simulink model "QuadArchitecture"  (R2026a)
settings: configuration reference "quad_config" (kept outside this file)
settings Model: DataDictionary=QuadData.sldd  PacingRate=4  Creator=The MathWorks, Inc.  LastModifiedBy=The MathWorks, Inc.
settings ConfigSetRef: SourceName=quad_config

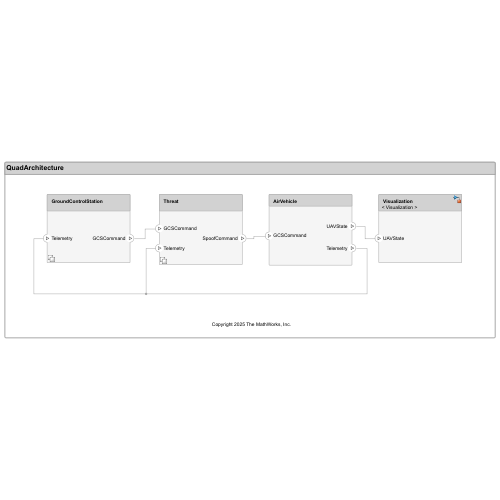
[thumbnail: Simulink's stored preview of the top-level diagram]
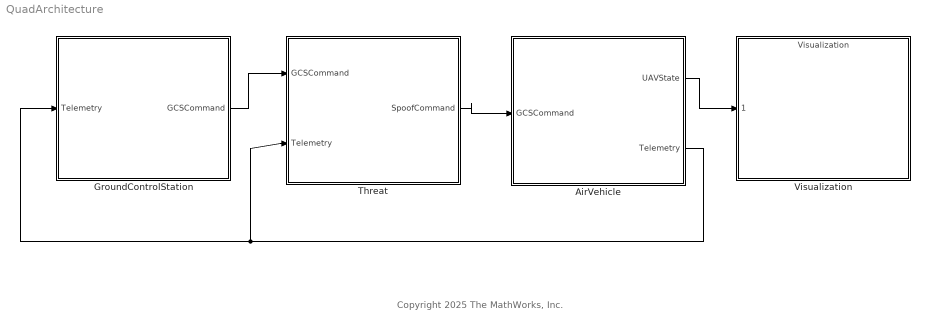
== system QuadArchitecture ==
  note: Copyright 2025 The MathWorks, Inc.
  AirVehicle : Subsystem
      settings: PortSchema="{\"entries\":[{\"content\":{\"headerSize\":26,\"margin\":15,\"minimumSpacing\":25,\"sides\":[{\"content\":{\"connectorIds\":[\"In1\"]},\"type\":\"ConnectorPlacement.EquallySpacedRectSide\",\"uuid\":\"972de20d-f328-4fd0-89f5-295843657512\"},{\"content\":{\"connectorIds\":[\"Out2\",\"Out1\"],\"side\":\"RIGHT\"},\"type\":\"ConnectorPlacement.EquallySpacedRectSide\",\"uuid\":\"134439da-fb85-42f0-a6e3-e26c335dbcbe\"},{\"content\":{\"side\":\"TOP\"},\"type\":\"ConnectorPlacement.EquallySpacedRectSide\",\"uuid\":\"868b2dd7-5d80-431a-bb16-a2f793ede056\"}]},\"type\":\"ConnectorPlacement.EquallySpacedConnector\",\"uuid\":\"adddc505-6cbf-480f-b95d-01cd6e84ae8d\"}],\"packageUris\":[\"http://schema.mathworks.com/mf0/Connector/R2020b\"],\"version\":\"1.0\"}"
  GroundControlStation : Subsystem  Variant=on  VariantControl=Choice
      settings: PortSchema="{\"entries\":[{\"content\":{\"headerSize\":38,\"margin\":15,\"minimumSpacing\":25,\"sides\":[{\"content\":{\"connectorIds\":[\"In1\"]},\"type\":\"ConnectorPlacement.EquallySpacedRectSide\",\"uuid\":\"7662a576-a240-432d-97be-55e19f57859a\"},{\"content\":{\"connectorIds\":[\"Out1\"],\"side\":\"RIGHT\"},\"type\":\"ConnectorPlacement.EquallySpacedRectSide\",\"uuid\":\"93b9fbbc-f8c4-4932-b9bb-3841cff066c6\"},{\"content\":{\"connectorIds\":[],\"side\":\"TOP\"},\"type\":\"ConnectorPlacement.EquallySpacedRectSide\",\"uuid\":\"5bdbe3e7-55b6-4275-a555-da2f215fbbe6\"}]},\"type\":\"ConnectorPlacement.EquallySpacedConnector\",\"uuid\":\"7fdcb0bb-8d60-4179-a2fb-32da7250d2ba\"}],\"packageUris\":[\"http://schema.mathworks.com/mf0/Connector/R2020b\"],\"version\":\"1.0\"}"
  Threat : Subsystem  Variant=on  VariantControl=Choice
      settings: PortSchema="{\"entries\":[{\"content\":{\"headerSize\":38,\"margin\":15,\"minimumSpacing\":25,\"sides\":[{\"content\":{\"connectorIds\":[\"In1\",\"In2\"]},\"type\":\"ConnectorPlacement.EquallySpacedRectSide\",\"uuid\":\"972de20d-f328-4fd0-89f5-295843657512\"},{\"content\":{\"connectorIds\":[\"Out1\"],\"side\":\"RIGHT\"},\"type\":\"ConnectorPlacement.EquallySpacedRectSide\",\"uuid\":\"134439da-fb85-42f0-a6e3-e26c335dbcbe\"},{\"content\":{\"side\":\"TOP\"},\"type\":\"ConnectorPlacement.EquallySpacedRectSide\",\"uuid\":\"868b2dd7-5d80-431a-bb16-a2f793ede056\"}]},\"type\":\"ConnectorPlacement.EquallySpacedConnector\",\"uuid\":\"adddc505-6cbf-480f-b95d-01cd6e84ae8d\"}],\"packageUris\":[\"http://schema.mathworks.com/mf0/Connector/R2020b\"],\"version\":\"1.0\"}"
  Visualization : ModelReference  ModelNameDialog=Visualization  SimulationMode=Normal  ModelReferenceVersion=11.4
      settings: PortSchema="{\"entries\":[{\"content\":{\"headerSize\":38,\"margin\":15,\"minimumSpacing\":25,\"sides\":[{\"content\":{\"connectorIds\":[\"In1\"]},\"type\":\"ConnectorPlacement.EquallySpacedRectSide\",\"uuid\":\"6721b7c2-8ab9-44e5-9ceb-8e1a3ee04589\"},{\"content\":{\"connectorIds\":[],\"side\":\"RIGHT\"},\"type\":\"ConnectorPlacement.EquallySpacedRectSide\",\"uuid\":\"3cd6ecf7-e51b-4f75-96cf-07e3d6ff229c\"},{\"content\":{\"connectorIds\":[],\"side\":\"TOP\"},\"type\":\"ConnectorPlacement.EquallySpacedRectSide\",\"uuid\":\"f91676ab-b0f6-405b-b8b9-c3171517e379\"}]},\"type\":\"ConnectorPlacement.EquallySpacedConnector\",\"uuid\":\"6f23ebeb-60da-469e-8f3b-5adae7c8af4f\"}],\"packageUris\":[\"http://schema.mathworks.com/mf0/Connector/R2020b\"],\"version\":\"1.0\"}"
  wires:
  AirVehicle/1(Telemetry) -> Threat/2(Telemetry), GroundControlStation/1(Telemetry)
  AirVehicle/2(UAVState) -> Visualization/1
  Threat/1(SpoofCommand) -> AirVehicle/1(GCSCommand)
  GroundControlStation/1(GCSCommand) -> Threat/1(GCSCommand)

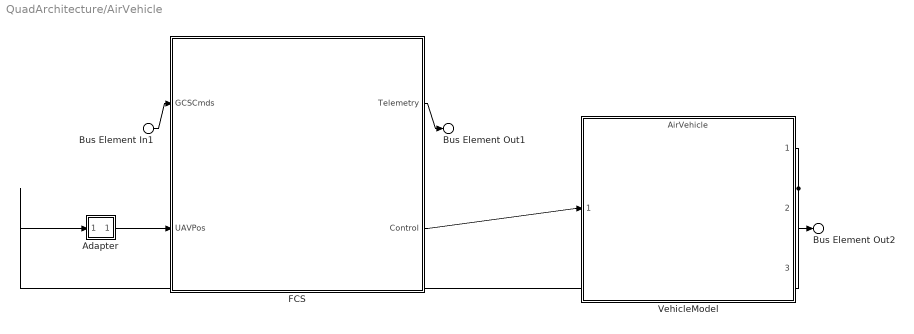
== system QuadArchitecture/AirVehicle ==
  Bus Element In1 : Inport  PortName=GCSCommand
  Adapter : Subsystem
      settings: PortSchema="{\"entries\":[{\"content\":{\"margin\":10,\"minimumSpacing\":15,\"sides\":[{\"content\":{\"connectorIds\":[\"In1\"]},\"type\":\"ConnectorPlacement.EquallySpacedRectSide\",\"uuid\":\"a2fff1cd-0e13-4741-b0cf-ef553acfd516\"},{\"content\":{\"connectorIds\":[\"Out1\"],\"side\":\"RIGHT\"},\"type\":\"ConnectorPlacement.EquallySpacedRectSide\",\"uuid\":\"37e44836-fd51-4d84-80b7-9025c833adfd\"},{\"content\":{\"connectorIds\":[],\"side\":\"TOP\"},\"type\":\"ConnectorPlacement.EquallySpacedRectSide\",\"uuid\":\"e6edc5e9-901f-4b36-8f7f-d0a35232da3b\"}]},\"type\":\"ConnectorPlacement.EquallySpacedConnector\",\"uuid\":\"83782042-2650-4988-9c4a-c1150f20d034\"}],\"packageUris\":[\"http://schema.mathworks.com/mf0/Connector/R2020b\"],\"version\":\"1.0\"}"
  FCS : Subsystem
      settings: PortSchema="{\"entries\":[{\"content\":{\"headerSize\":26,\"margin\":15,\"minimumSpacing\":25,\"sides\":[{\"content\":{\"connectorIds\":[\"In1\",\"In2\"]},\"type\":\"ConnectorPlacement.EquallySpacedRectSide\",\"uuid\":\"c19c5851-94a8-41ae-97b5-784b7360f27c\"},{\"content\":{\"connectorIds\":[\"Out1\",\"Out2\"],\"side\":\"RIGHT\"},\"type\":\"ConnectorPlacement.EquallySpacedRectSide\",\"uuid\":\"5a0e265f-6421-459c-9b38-1ace018e6962\"},{\"content\":{\"side\":\"TOP\"},\"type\":\"ConnectorPlacement.EquallySpacedRectSide\",\"uuid\":\"afc92b11-75c7-4a4a-94ab-c0816f6717ed\"}]},\"type\":\"ConnectorPlacement.EquallySpacedConnector\",\"uuid\":\"e74c21e7-420a-47a8-adb7-493ac11b1149\"}],\"packageUris\":[\"http://schema.mathworks.com/mf0/Connector/R2020b\"],\"version\":\"1.0\"}"
  VehicleModel : ModelReference  ModelNameDialog=AirVehicle  ModelReferenceVersion=12.4
      settings: PortSchema="{\"entries\":[{\"content\":{\"headerSize\":38,\"margin\":15,\"minimumSpacing\":25,\"sides\":[{\"content\":{\"connectorIds\":[\"In1\"]},\"type\":\"ConnectorPlacement.EquallySpacedRectSide\",\"uuid\":\"972de20d-f328-4fd0-89f5-295843657512\"},{\"content\":{\"connectorIds\":[\"Out1\",\"Out2\",\"Out3\"],\"side\":\"RIGHT\"},\"type\":\"ConnectorPlacement.EquallySpacedRectSide\",\"uuid\":\"134439da-fb85-42f0-a6e3-e26c335dbcbe\"},{\"content\":{\"side\":\"TOP\"},\"type\":\"ConnectorPlacement.EquallySpacedRectSide\",\"uuid\":\"868b2dd7-5d80-431a-bb16-a2f793ede056\"}]},\"type\":\"ConnectorPlacement.EquallySpacedConnector\",\"uuid\":\"adddc505-6cbf-480f-b95d-01cd6e84ae8d\"}],\"packageUris\":[\"http://schema.mathworks.com/mf0/Connector/R2020b\"],\"version\":\"1.0\"}"
  Bus Element Out1 : Outport  PortName=Telemetry
  Bus Element Out2 : Outport  Port=2  PortName=UAVState
  wires:
  FCS/1(Telemetry) -> Bus Element Out1/1
  VehicleModel/1 -> Bus Element Out2/1, Adapter/1(In)
  FCS/2(Control) -> VehicleModel/1
  Adapter/1(UAVPos) -> FCS/2(UAVPos)
  Bus Element In1/1 -> FCS/1(GCSCmds)

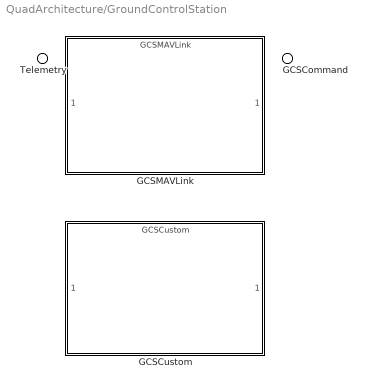
== system QuadArchitecture/GroundControlStation ==
  Telemetry : Inport
  GCSCustom : ModelReference  ModelNameDialog=GCSCustom  SimulationMode=Normal  VariantControl=varComms == 2  ModelReferenceVersion=12.2
      settings: PortSchema="{\"entries\":[{\"content\":{\"headerSize\":38,\"margin\":15,\"minimumSpacing\":25,\"sides\":[{\"content\":{\"connectorIds\":[\"In1\"]},\"type\":\"ConnectorPlacement.EquallySpacedRectSide\",\"uuid\":\"972de20d-f328-4fd0-89f5-295843657512\"},{\"content\":{\"connectorIds\":[\"Out1\"],\"side\":\"RIGHT\"},\"type\":\"ConnectorPlacement.EquallySpacedRectSide\",\"uuid\":\"134439da-fb85-42f0-a6e3-e26c335dbcbe\"},{\"content\":{\"connectorIds\":[],\"side\":\"TOP\"},\"type\":\"ConnectorPlacement.EquallySpacedRectSide\",\"uuid\":\"868b2dd7-5d80-431a-bb16-a2f793ede056\"}]},\"type\":\"ConnectorPlacement.EquallySpacedConnector\",\"uuid\":\"adddc505-6cbf-480f-b95d-01cd6e84ae8d\"}],\"packageUris\":[\"http://schema.mathworks.com/mf0/Connector/R2020b\"],\"version\":\"1.0\"}"
  GCSMAVLink : ModelReference  ModelNameDialog=GCSMAVLink  SimulationMode=Normal  VariantControl=varComms == 1  ModelReferenceVersion=12.4
      settings: PortSchema="{\"entries\":[{\"content\":{\"headerSize\":38,\"margin\":15,\"minimumSpacing\":25,\"sides\":[{\"content\":{\"connectorIds\":[\"In1\"]},\"type\":\"ConnectorPlacement.EquallySpacedRectSide\",\"uuid\":\"7662a576-a240-432d-97be-55e19f57859a\"},{\"content\":{\"connectorIds\":[\"Out1\"],\"side\":\"RIGHT\"},\"type\":\"ConnectorPlacement.EquallySpacedRectSide\",\"uuid\":\"93b9fbbc-f8c4-4932-b9bb-3841cff066c6\"},{\"content\":{\"connectorIds\":[],\"side\":\"TOP\"},\"type\":\"ConnectorPlacement.EquallySpacedRectSide\",\"uuid\":\"5bdbe3e7-55b6-4275-a555-da2f215fbbe6\"}]},\"type\":\"ConnectorPlacement.EquallySpacedConnector\",\"uuid\":\"7fdcb0bb-8d60-4179-a2fb-32da7250d2ba\"}],\"packageUris\":[\"http://schema.mathworks.com/mf0/Connector/R2020b\"],\"version\":\"1.0\"}"
  GCSCommand : Outport  OutDataTypeStr=Bus: GCSCmds

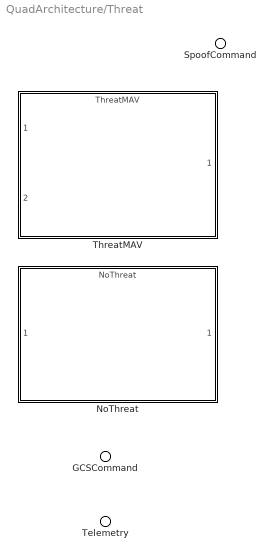
== system QuadArchitecture/Threat ==
  GCSCommand : Inport
  Telemetry : Inport  Port=2
  NoThreat : ModelReference  ModelNameDialog=NoThreat  SimulationMode=Normal  VariantControl=varThreat == 0  ModelReferenceVersion=2.0
      settings: PortSchema="{\"entries\":[{\"content\":{\"headerSize\":38,\"margin\":15,\"minimumSpacing\":25,\"sides\":[{\"content\":{\"connectorIds\":[\"In1\"]},\"type\":\"ConnectorPlacement.EquallySpacedRectSide\",\"uuid\":\"e9d8ad3e-caa9-432a-b411-be5fd036b273\"},{\"content\":{\"connectorIds\":[\"Out1\"],\"side\":\"RIGHT\"},\"type\":\"ConnectorPlacement.EquallySpacedRectSide\",\"uuid\":\"3984a8dd-9d03-4219-b4db-e54bb042947b\"},{\"content\":{\"side\":\"TOP\"},\"type\":\"ConnectorPlacement.EquallySpacedRectSide\",\"uuid\":\"6391b23f-1c48-490d-9fba-fd835ec6a9a7\"}]},\"type\":\"ConnectorPlacement.EquallySpacedConnector\",\"uuid\":\"c696faa4-67d5-4608-8425-39d05734b4d9\"}],\"packageUris\":[\"http://schema.mathworks.com/mf0/Connector/R2020b\"],\"version\":\"1.0\"}"
  ThreatMAV : ModelReference  ModelNameDialog=ThreatMAV  SimulationMode=Normal  VariantControl=varThreat == 1  ModelReferenceVersion=12.4
      settings: PortSchema="{\"entries\":[{\"content\":{\"headerSize\":38,\"margin\":15,\"minimumSpacing\":25,\"sides\":[{\"content\":{\"connectorIds\":[\"In1\",\"In2\"]},\"type\":\"ConnectorPlacement.EquallySpacedRectSide\",\"uuid\":\"972de20d-f328-4fd0-89f5-295843657512\"},{\"content\":{\"connectorIds\":[\"Out1\"],\"side\":\"RIGHT\"},\"type\":\"ConnectorPlacement.EquallySpacedRectSide\",\"uuid\":\"134439da-fb85-42f0-a6e3-e26c335dbcbe\"},{\"content\":{\"connectorIds\":[],\"side\":\"TOP\"},\"type\":\"ConnectorPlacement.EquallySpacedRectSide\",\"uuid\":\"868b2dd7-5d80-431a-bb16-a2f793ede056\"}]},\"type\":\"ConnectorPlacement.EquallySpacedConnector\",\"uuid\":\"adddc505-6cbf-480f-b95d-01cd6e84ae8d\"}],\"packageUris\":[\"http://schema.mathworks.com/mf0/Connector/R2020b\"],\"version\":\"1.0\"}"
  SpoofCommand : Outport  OutDataTypeStr=Bus: GCSCmds

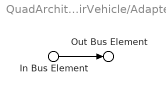
== system QuadArchitecture/AirVehicle/Adapter ==
  In Bus Element : Inport  PortName=In
  Out Bus Element : Outport  PortName=UAVPos
  wires:
  In Bus Element/1 -> Out Bus Element/1

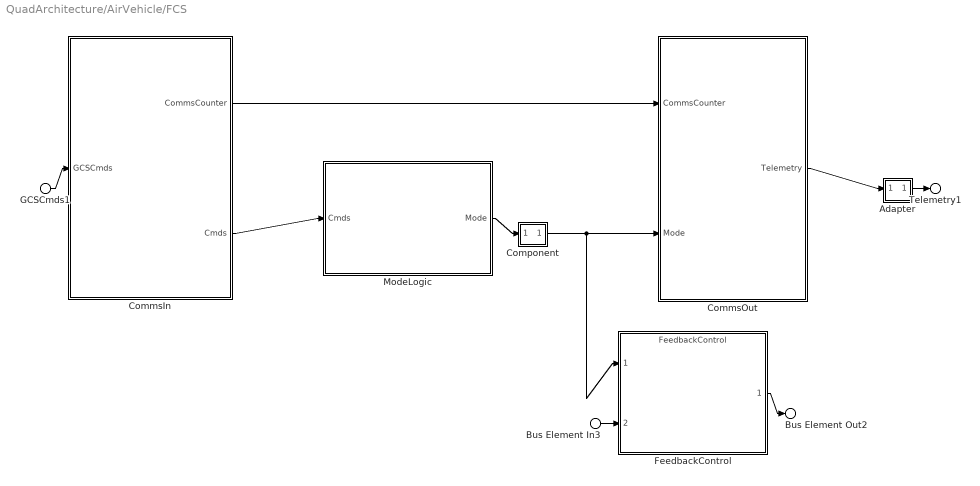
== system QuadArchitecture/AirVehicle/FCS ==
  GCSCmds1 : Inport  PortName=GCSCmds
  Bus Element In3 : Inport  Port=2  PortName=UAVPos
  Adapter : Subsystem
      settings: PortSchema="{\"entries\":[{\"content\":{\"margin\":10,\"minimumSpacing\":15,\"sides\":[{\"content\":{\"connectorIds\":[\"In1\"]},\"type\":\"ConnectorPlacement.EquallySpacedRectSide\",\"uuid\":\"54e91e87-63c7-4e3e-b7b9-664b6d97de79\"},{\"content\":{\"connectorIds\":[\"Out1\"],\"side\":\"RIGHT\"},\"type\":\"ConnectorPlacement.EquallySpacedRectSide\",\"uuid\":\"42371d78-e1ed-48f1-9b63-a93cba4f2c4a\"},{\"content\":{\"side\":\"TOP\"},\"type\":\"ConnectorPlacement.EquallySpacedRectSide\",\"uuid\":\"1916e499-1a19-4cfc-bc1b-e5fae3753eb5\"},{\"content\":{\"side\":\"BOTTOM\"},\"type\":\"ConnectorPlacement.EquallySpacedRectSide\",\"uuid\":\"be41fb80-b3af-48dd-88cd-2631e5331a74\"},{\"content\":{\"side\":\"HIDDEN\"},\"type\":\"ConnectorPlacement.EquallySpacedRectSide\",\"uuid\":\"3c256238-c293-40f1-b4b8-16721d7c0eb8\"}]},\"type\":\"ConnectorPlacement.EquallySpacedConnector\",\"uuid\":\"450fde28-8b10-4341-ad28-487e19ca1e28\"}],\"packageUris\":[\"http://schema.mathworks.com/mf0/Connector/R2020b\"],\"version\":\"1.0\"}"
  CommsIn : Subsystem  Variant=on  VariantControl=Choice
      settings: PortSchema="{\"entries\":[{\"content\":{\"headerSize\":38,\"margin\":15,\"minimumSpacing\":25,\"sides\":[{\"content\":{\"connectorIds\":[\"In1\"]},\"type\":\"ConnectorPlacement.EquallySpacedRectSide\",\"uuid\":\"972de20d-f328-4fd0-89f5-295843657512\"},{\"content\":{\"connectorIds\":[\"Out1\",\"Out2\"],\"side\":\"RIGHT\"},\"type\":\"ConnectorPlacement.EquallySpacedRectSide\",\"uuid\":\"134439da-fb85-42f0-a6e3-e26c335dbcbe\"},{\"content\":{\"connectorIds\":[],\"side\":\"TOP\"},\"type\":\"ConnectorPlacement.EquallySpacedRectSide\",\"uuid\":\"868b2dd7-5d80-431a-bb16-a2f793ede056\"}]},\"type\":\"ConnectorPlacement.EquallySpacedConnector\",\"uuid\":\"adddc505-6cbf-480f-b95d-01cd6e84ae8d\"}],\"packageUris\":[\"http://schema.mathworks.com/mf0/Connector/R2020b\"],\"version\":\"1.0\"}"
  CommsOut : Subsystem  Variant=on  VariantControl=Choice
      settings: PortSchema="{\"entries\":[{\"content\":{\"headerSize\":38,\"margin\":15,\"minimumSpacing\":25,\"sides\":[{\"content\":{\"connectorIds\":[\"In1\",\"In2\"]},\"type\":\"ConnectorPlacement.EquallySpacedRectSide\",\"uuid\":\"972de20d-f328-4fd0-89f5-295843657512\"},{\"content\":{\"connectorIds\":[\"Out1\"],\"side\":\"RIGHT\"},\"type\":\"ConnectorPlacement.EquallySpacedRectSide\",\"uuid\":\"134439da-fb85-42f0-a6e3-e26c335dbcbe\"},{\"content\":{\"connectorIds\":[],\"side\":\"TOP\"},\"type\":\"ConnectorPlacement.EquallySpacedRectSide\",\"uuid\":\"868b2dd7-5d80-431a-bb16-a2f793ede056\"}]},\"type\":\"ConnectorPlacement.EquallySpacedConnector\",\"uuid\":\"adddc505-6cbf-480f-b95d-01cd6e84ae8d\"}],\"packageUris\":[\"http://schema.mathworks.com/mf0/Connector/R2020b\"],\"version\":\"1.0\"}"
  Component : Subsystem
      settings: PortSchema="{\"entries\":[{\"content\":{\"margin\":10,\"minimumSpacing\":15,\"sides\":[{\"content\":{\"connectorIds\":[\"In1\"]},\"type\":\"ConnectorPlacement.EquallySpacedRectSide\",\"uuid\":\"17bee697-cd3a-4e06-942d-dac2ea0385a6\"},{\"content\":{\"connectorIds\":[\"Out1\"],\"side\":\"RIGHT\"},\"type\":\"ConnectorPlacement.EquallySpacedRectSide\",\"uuid\":\"6d1b1a8d-a046-48b6-94d3-1fa2831d6db3\"},{\"content\":{\"side\":\"TOP\"},\"type\":\"ConnectorPlacement.EquallySpacedRectSide\",\"uuid\":\"a053ff8f-e369-4dd3-abbb-f0419cd0218c\"}]},\"type\":\"ConnectorPlacement.EquallySpacedConnector\",\"uuid\":\"3ac54abc-4df1-48cf-8f38-e2b144d46944\"}],\"packageUris\":[\"http://schema.mathworks.com/mf0/Connector/R2020b\"],\"version\":\"1.0\"}"
  FeedbackControl : ModelReference  ModelNameDialog=FeedbackControl  SimulationMode=Normal  ModelReferenceVersion=8.3
      settings: PortSchema="{\"entries\":[{\"content\":{\"headerSize\":38,\"margin\":15,\"minimumSpacing\":25,\"sides\":[{\"content\":{\"connectorIds\":[\"In1\",\"In2\"]},\"type\":\"ConnectorPlacement.EquallySpacedRectSide\",\"uuid\":\"a2fff1cd-0e13-4741-b0cf-ef553acfd516\"},{\"content\":{\"connectorIds\":[\"Out1\"],\"side\":\"RIGHT\"},\"type\":\"ConnectorPlacement.EquallySpacedRectSide\",\"uuid\":\"37e44836-fd51-4d84-80b7-9025c833adfd\"},{\"content\":{\"side\":\"TOP\"},\"type\":\"ConnectorPlacement.EquallySpacedRectSide\",\"uuid\":\"e6edc5e9-901f-4b36-8f7f-d0a35232da3b\"}]},\"type\":\"ConnectorPlacement.EquallySpacedConnector\",\"uuid\":\"83782042-2650-4988-9c4a-c1150f20d034\"}],\"packageUris\":[\"http://schema.mathworks.com/mf0/Connector/R2020b\"],\"version\":\"1.0\"}"
  ModeLogic : Stateflow chart  TreatAsAtomicUnit=on
      settings: PortSchema="{\"entries\":[{\"content\":{\"headerSize\":26,\"margin\":15,\"minimumSpacing\":25,\"sides\":[{\"content\":{\"connectorIds\":[\"In1\"]},\"type\":\"ConnectorPlacement.EquallySpacedRectSide\",\"uuid\":\"a2fff1cd-0e13-4741-b0cf-ef553acfd516\"},{\"content\":{\"connectorIds\":[\"Out1\"],\"side\":\"RIGHT\"},\"type\":\"ConnectorPlacement.EquallySpacedRectSide\",\"uuid\":\"37e44836-fd51-4d84-80b7-9025c833adfd\"},{\"content\":{\"connectorIds\":[],\"side\":\"TOP\"},\"type\":\"ConnectorPlacement.EquallySpacedRectSide\",\"uuid\":\"e6edc5e9-901f-4b36-8f7f-d0a35232da3b\"}]},\"type\":\"ConnectorPlacement.EquallySpacedConnector\",\"uuid\":\"83782042-2650-4988-9c4a-c1150f20d034\"}],\"packageUris\":[\"http://schema.mathworks.com/mf0/Connector/R2020b\"],\"version\":\"1.0\"}"
  Telemetry1 : Outport  PortName=Telemetry
  Bus Element Out2 : Outport  Port=2  PortName=Control
  wires:
  CommsIn/1(CommsCounter) -> CommsOut/1(CommsCounter)
  CommsIn/2(Cmds) -> ModeLogic/1(Cmds)
  GCSCmds1/1 -> CommsIn/1(GCSCmds)
  FeedbackControl/1 -> Bus Element Out2/1
  Bus Element In3/1 -> FeedbackControl/2
  ModeLogic/1(Mode) -> Component/1(In)
  Component/1(Out) -> FeedbackControl/1, CommsOut/2(Mode)
  CommsOut/1(Telemetry) -> Adapter/1(TelemetryIn)
  Adapter/1(Telemetry) -> Telemetry1/1

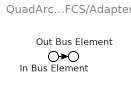
== system QuadArchitecture/AirVehicle/FCS/Adapter ==
  In Bus Element : Inport  PortName=TelemetryIn
  Out Bus Element : Outport  PortName=Telemetry
  wires:
  In Bus Element/1 -> Out Bus Element/1

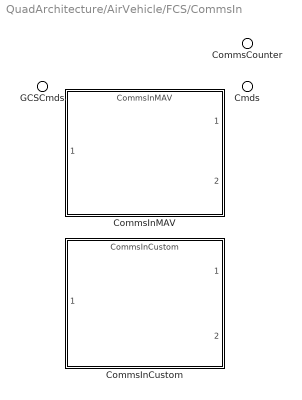
== system QuadArchitecture/AirVehicle/FCS/CommsIn ==
  GCSCmds : Inport  OutDataTypeStr=Bus: GCSCmds
  CommsInCustom : ModelReference  ModelNameDialog=CommsInCustom  SimulationMode=Normal  VariantControl=varComms == 2  ModelReferenceVersion=8.0
      settings: PortSchema="{\"entries\":[{\"content\":{\"headerSize\":38,\"margin\":15,\"minimumSpacing\":25,\"sides\":[{\"content\":{\"connectorIds\":[\"In1\"]},\"type\":\"ConnectorPlacement.EquallySpacedRectSide\",\"uuid\":\"972de20d-f328-4fd0-89f5-295843657512\"},{\"content\":{\"connectorIds\":[\"Out1\",\"Out2\"],\"side\":\"RIGHT\"},\"type\":\"ConnectorPlacement.EquallySpacedRectSide\",\"uuid\":\"134439da-fb85-42f0-a6e3-e26c335dbcbe\"},{\"content\":{\"connectorIds\":[],\"side\":\"TOP\"},\"type\":\"ConnectorPlacement.EquallySpacedRectSide\",\"uuid\":\"868b2dd7-5d80-431a-bb16-a2f793ede056\"}]},\"type\":\"ConnectorPlacement.EquallySpacedConnector\",\"uuid\":\"adddc505-6cbf-480f-b95d-01cd6e84ae8d\"}],\"packageUris\":[\"http://schema.mathworks.com/mf0/Connector/R2020b\"],\"version\":\"1.0\"}"
  CommsInMAV : ModelReference  ModelNameDialog=CommsInMAV  SimulationMode=Normal  VariantControl=varComms == 1  ModelReferenceVersion=8.1
      settings: PortSchema="{\"entries\":[{\"content\":{\"headerSize\":38,\"margin\":15,\"minimumSpacing\":25,\"sides\":[{\"content\":{\"connectorIds\":[\"In1\"]},\"type\":\"ConnectorPlacement.EquallySpacedRectSide\",\"uuid\":\"972de20d-f328-4fd0-89f5-295843657512\"},{\"content\":{\"connectorIds\":[\"Out1\",\"Out2\"],\"side\":\"RIGHT\"},\"type\":\"ConnectorPlacement.EquallySpacedRectSide\",\"uuid\":\"134439da-fb85-42f0-a6e3-e26c335dbcbe\"},{\"content\":{\"connectorIds\":[],\"side\":\"TOP\"},\"type\":\"ConnectorPlacement.EquallySpacedRectSide\",\"uuid\":\"868b2dd7-5d80-431a-bb16-a2f793ede056\"}]},\"type\":\"ConnectorPlacement.EquallySpacedConnector\",\"uuid\":\"adddc505-6cbf-480f-b95d-01cd6e84ae8d\"}],\"packageUris\":[\"http://schema.mathworks.com/mf0/Connector/R2020b\"],\"version\":\"1.0\"}"
  CommsCounter : Outport
  Cmds : Outport  Port=2  OutDataTypeStr=Bus: Cmds

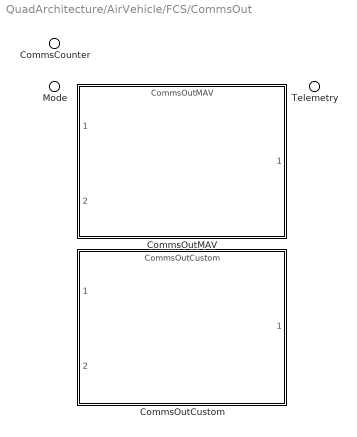
== system QuadArchitecture/AirVehicle/FCS/CommsOut ==
  CommsCounter : Inport
  Mode : Inport  Port=2
  CommsOutCustom : ModelReference  ModelNameDialog=CommsOutCustom  SimulationMode=Normal  VariantControl=varComms == 2  ModelReferenceVersion=8.0
      settings: PortSchema="{\"entries\":[{\"content\":{\"headerSize\":38,\"margin\":15,\"minimumSpacing\":25,\"sides\":[{\"content\":{\"connectorIds\":[\"In1\",\"In2\"]},\"type\":\"ConnectorPlacement.EquallySpacedRectSide\",\"uuid\":\"972de20d-f328-4fd0-89f5-295843657512\"},{\"content\":{\"connectorIds\":[\"Out1\"],\"side\":\"RIGHT\"},\"type\":\"ConnectorPlacement.EquallySpacedRectSide\",\"uuid\":\"134439da-fb85-42f0-a6e3-e26c335dbcbe\"},{\"content\":{\"connectorIds\":[],\"side\":\"TOP\"},\"type\":\"ConnectorPlacement.EquallySpacedRectSide\",\"uuid\":\"868b2dd7-5d80-431a-bb16-a2f793ede056\"}]},\"type\":\"ConnectorPlacement.EquallySpacedConnector\",\"uuid\":\"adddc505-6cbf-480f-b95d-01cd6e84ae8d\"}],\"packageUris\":[\"http://schema.mathworks.com/mf0/Connector/R2020b\"],\"version\":\"1.0\"}"
  CommsOutMAV : ModelReference  ModelNameDialog=CommsOutMAV  SimulationMode=Normal  VariantControl=varComms == 1  ModelReferenceVersion=8.0
      settings: PortSchema="{\"entries\":[{\"content\":{\"headerSize\":38,\"margin\":15,\"minimumSpacing\":25,\"sides\":[{\"content\":{\"connectorIds\":[\"In1\",\"In2\"]},\"type\":\"ConnectorPlacement.EquallySpacedRectSide\",\"uuid\":\"972de20d-f328-4fd0-89f5-295843657512\"},{\"content\":{\"connectorIds\":[\"Out1\"],\"side\":\"RIGHT\"},\"type\":\"ConnectorPlacement.EquallySpacedRectSide\",\"uuid\":\"134439da-fb85-42f0-a6e3-e26c335dbcbe\"},{\"content\":{\"connectorIds\":[],\"side\":\"TOP\"},\"type\":\"ConnectorPlacement.EquallySpacedRectSide\",\"uuid\":\"868b2dd7-5d80-431a-bb16-a2f793ede056\"}]},\"type\":\"ConnectorPlacement.EquallySpacedConnector\",\"uuid\":\"adddc505-6cbf-480f-b95d-01cd6e84ae8d\"}],\"packageUris\":[\"http://schema.mathworks.com/mf0/Connector/R2020b\"],\"version\":\"1.0\"}"
  Telemetry : Outport

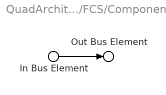
== system QuadArchitecture/AirVehicle/FCS/Component ==
  In Bus Element : Inport  PortName=In
  Out Bus Element : Outport  PortName=Out
  wires:
  In Bus Element/1 -> Out Bus Element/1

== stateflow chart QuadArchitecture/AirVehicle/FCS/ModeLogic ==
  note: Mode
      | ---------
      |
      | 0: OnGround
      | 1: Flying
      | 2: Landing
      | 3: EmergencyOff
  state OnGround
    en: Mode = 0;
  state EmergencyOff
    en: Mode = 3;
  state Flying
    en: Mode = 1;
  state Landing
    en: Mode = 2;
  (default) -> OnGround
  OnGround -> Flying : [Cmds.Takeoff]
  Flying -> (junction 5) [order 2]
  Flying -> Landing [order 1] : [Cmds.Land]
  (junction 5) -> EmergencyOff : [Cmds.EmergencyOff]
  Landing -> (junction 5)
  data: Cmds input Bus: Cmds; Mode output uint8
